simulink model "clutch"  (R2020a)
settings: Solver=ode3  StartTime=0.0  StopTime=30  FixedStep=1e-3  RelTol=1e-3
undefined symbols (not defined in the file or in its folder): be, bv, Ie, Iv, Kd, Ki, Kp, kv, Tclmax
libraries: simulink x2
settings Model: Creator=User  LastModifiedBy=User
settings SolverCC: ZeroCrossAlgorithm=Adaptive
settings DebuggingCC: IgnoredZcDiagnostic=none

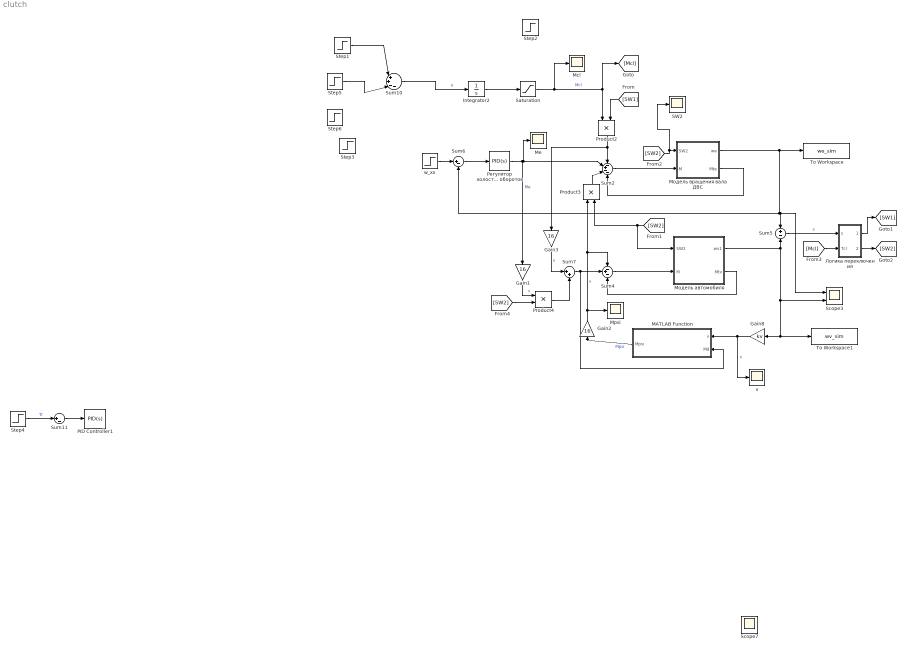
== system clutch ==
  Gain1 : Gain  Gain=16
  Gain2 : Gain  Gain=16
  Gain3 : Gain  Gain=16
  Gain8 : Gain  Gain=kv
  Integrator2 : Integrator
  MATLAB Function : MATLAB Function  TreatAsAtomicUnit=on
  Mcl : Scope
  Me : Scope
  Mpsi : Scope
  PID Controller1 : simulink/Continuous/PID Controller  Controller=PID  Form=Parallel  TimeDomain=Continuous-time  UseExternalTs=off  SampleTime=-1  IntegratorMethod=Forward Euler  FilterMethod=Forward Euler  ControllerParametersSource=internal  P=Kp  I=Ki  D=Kd  UseFilter=on  N=100  TunerSelectOption=Transfer Function Based (PID Tuner App)  InitialConditionSource=internal  InitialConditionForIntegrator=0  InitialConditionForFilter=0  DifferentiatorICPrevScaledInput=0  ExternalReset=none  TrackingMode=off  Kt=1  LimitOutput=off  UpperSaturationLimit=inf  LowerSaturationLimit=0  LinearizeAsGain=on  AntiWindupMode=none  Kb=1  POutMin=[]  POutMax=[]  IOutMin=[]  IOutMax=[]  DOutMin=[]  DOutMax=[]  NOutMin=[]  NOutMax=[]  SumOutMin=[]  SumOutMax=[]  SaturationOutMin=[]  SaturationOutMax=[]  PParamMin=[]  PParamMax=[]  IParamMin=[]  IParamMax=[]  DParamMin=[]  DParamMax=[]  NParamMin=[]  NParamMax=[]  KbParamMin=[]  KbParamMax=[]  KtParamMin=[]  KtParamMax=[]  KbOutMin=[]  KbOutMax=[]  KtOutMin=[]  KtOutMax=[]  IntegratorOutMin=[]  IntegratorOutMax=[]  FilterOutMin=[]  FilterOutMax=[]  SumI1OutMin=[]  SumI1OutMax=[]  SumI2OutMin=[]  SumI2OutMax=[]  SumI3OutMin=[]  SumI3OutMax=[]  SumI4OutMin=[]  SumI4OutMax=[]  SumDOutMin=[]  SumDOutMax=[]  DifferentiatorOutMin=[]  DifferentiatorOutMax=[]  FilterDiffOutCoefMin=[]  FilterDiffOutCoefMax=[]  ReciprocalOutMin=[]  ReciprocalOutMax=[]  SumDenOutMin=[]  SumDenOutMax=[]  SumNumOutMin=[]  SumNumOutMax=[]  DivideOutMin=[]  DivideOutMax=[]  UdiffTsProdOutMin=[]  UdiffTsProdOutMax=[]  NTsProdOutMin=[]  NTsProdOutMax=[]  UintegralTsProdOutMin=[]  UintegralTsProdOutMax=[]  UngainTsProdOutMin=[]  UngainTsProdOutMax=[]  IntegratorContinuousStateAttributes=''  IntegratorStateMustResolveToSignalObject=off  IntegratorRTWStateStorageClass=Auto  FilterContinuousStateAttributes=''  FilterStateMustResolveToSignalObject=off  FilterRTWStateStorageClass=Auto  ParallelPVariant=InternalParameters  IdealPVariant=Disabled  IVariant=InternalParameters  DVariant=InternalParameters  IntegratorVariant=Continuous  SatVariant=Disabled  AWVariant=Passthrough  PCopyVariant=Disabled  TRVariant=Disabled  FdbkBlocksVariant=Forward  IdealPFdbkVariant=Disabled  SatFdbkVariant=Disabled  DerivativeFilterVariant=ContFilter  NVariant=InternalParameters  NCopyVariant=Disabled  FilterICVariant=InternalICsFilter  IntegratorICVariant=InternalICs  ExternalResetVariant=Disabled  TRSumVariant=Passthrough  SumFdbkVariant=Disabled  SumVariant=Sum_PID  TsampFilterVariant=InternalTs  TsampNgainVariant=Passthrough  TsampIntegralVariant=Passthrough
  Product2 : Product
  Product3 : Product
  Product4 : Product
  SW2 : Scope
  Saturation : Saturate  UpperLimit=Tclmax  LowerLimit=0
  Scope3 : Scope  NumInputPorts=2
  Scope7 : Scope
  Step1 : Step  Time=2.9  After=50/2  SampleTime=0
  Step2 : Step  Time=2.9  After=50/2  SampleTime=0
  Step3 : Step  Time=17  After=100/1  SampleTime=0
  Step4 : Step  Time=5  After=6  SampleTime=0
  Step5 : Step  Time=10  After=1000/1  SampleTime=0
  Step6 : Step  Time=12  After=100/1  SampleTime=0
  Sum10 : Sum  Inputs=|++--
  Sum11 : Sum  Inputs=|+-
  Sum2 : Sum  Inputs=-+--
  Sum4 : Sum  Inputs=-+-
  Sum5 : Sum  Inputs=+|-
  Sum6 : Sum  Inputs=|+-
  Sum7 : Sum  Inputs=|++
  To Workspace : ToWorkspace  VariableName=we_sim  SaveFormat=Timeseries  SampleTime=-1
  To Workspace1 : ToWorkspace  VariableName=wv_sim  SaveFormat=Timeseries  SampleTime=-1
  v : Scope
  w_xx : Step  Time=10  Before=750  After=750  SampleTime=0
  Логика переключения : Subsystem
  Модель автомобиля : Subsystem
  Модель вращения вала ДВС : Subsystem
  Регулятор холостых оборотов : simulink/Continuous/PID Controller  Controller=PID  Form=Parallel  TimeDomain=Continuous-time  UseExternalTs=off  SampleTime=-1  IntegratorMethod=Forward Euler  FilterMethod=Forward Euler  ControllerParametersSource=internal  P=0.5  I=1  D=0  UseFilter=on  N=100  TunerSelectOption=Transfer Function Based (PID Tuner App)  InitialConditionSource=internal  InitialConditionForIntegrator=20  InitialConditionForFilter=0  DifferentiatorICPrevScaledInput=0  ExternalReset=none  TrackingMode=off  Kt=1  LimitOutput=off  UpperSaturationLimit=inf  LowerSaturationLimit=0  LinearizeAsGain=on  AntiWindupMode=none  Kb=1  POutMin=[]  POutMax=[]  IOutMin=[]  IOutMax=[]  DOutMin=[]  DOutMax=[]  NOutMin=[]  NOutMax=[]  SumOutMin=[]  SumOutMax=[]  SaturationOutMin=[]  SaturationOutMax=[]  PParamMin=[]  PParamMax=[]  IParamMin=[]  IParamMax=[]  DParamMin=[]  DParamMax=[]  NParamMin=[]  NParamMax=[]  KbParamMin=[]  KbParamMax=[]  KtParamMin=[]  KtParamMax=[]  KbOutMin=[]  KbOutMax=[]  KtOutMin=[]  KtOutMax=[]  IntegratorOutMin=[]  IntegratorOutMax=[]  FilterOutMin=[]  FilterOutMax=[]  SumI1OutMin=[]  SumI1OutMax=[]  SumI2OutMin=[]  SumI2OutMax=[]  SumI3OutMin=[]  SumI3OutMax=[]  SumI4OutMin=[]  SumI4OutMax=[]  SumDOutMin=[]  SumDOutMax=[]  DifferentiatorOutMin=[]  DifferentiatorOutMax=[]  FilterDiffOutCoefMin=[]  FilterDiffOutCoefMax=[]  ReciprocalOutMin=[]  ReciprocalOutMax=[]  SumDenOutMin=[]  SumDenOutMax=[]  SumNumOutMin=[]  SumNumOutMax=[]  DivideOutMin=[]  DivideOutMax=[]  UdiffTsProdOutMin=[]  UdiffTsProdOutMax=[]  NTsProdOutMin=[]  NTsProdOutMax=[]  UintegralTsProdOutMin=[]  UintegralTsProdOutMax=[]  UngainTsProdOutMin=[]  UngainTsProdOutMax=[]  IntegratorContinuousStateAttributes=''  IntegratorStateMustResolveToSignalObject=off  IntegratorRTWStateStorageClass=Auto  FilterContinuousStateAttributes=''  FilterStateMustResolveToSignalObject=off  FilterRTWStateStorageClass=Auto  ParallelPVariant=InternalParameters  IdealPVariant=Disabled  IVariant=InternalParameters  DVariant=InternalParameters  IntegratorVariant=Continuous  SatVariant=Disabled  AWVariant=Passthrough  PCopyVariant=Disabled  TRVariant=Disabled  FdbkBlocksVariant=Forward  IdealPFdbkVariant=Disabled  SatFdbkVariant=Disabled  DerivativeFilterVariant=ContFilter  NVariant=InternalParameters  NCopyVariant=Disabled  FilterICVariant=InternalICsFilter  IntegratorICVariant=InternalICs  ExternalResetVariant=Disabled  TRSumVariant=Passthrough  SumFdbkVariant=Disabled  SumVariant=Sum_PID  TsampFilterVariant=InternalTs  TsampNgainVariant=Passthrough  TsampIntegralVariant=Passthrough
  wires:
  Sum10/1 -> Integrator2/1  "u"
  Product3/1 -> Sum2/3
  ? -> Sum11/2
  [Mcl] -> Логика переключения/2(Tcl)
  Модель автомобиля/1(wv1) -> Scope3/2, To Workspace1/1, Gain8/1, Sum5/2
  Sum4/1 -> Модель автомобиля/2(M)
  Модель вращения вала ДВС/1(we) -> Scope3/1, Sum5/1, Sum6/2, To Workspace/1
  [SW2] -> Модель автомобиля/1(SW2), Product3/2
  Saturation/1 -> Mcl/1, [Mcl], Product2/1  "Mcl"
  Sum2/1 -> Модель вращения вала ДВС/2(M)
  MATLAB Function/1(Mpsi) -> Gain2/1  "Mpsi"
  Sum11/1 -> PID Controller1/1
  [SW1] -> Product2/2
  Gain8/1 -> MATLAB Function/1(v), v/1  "v"
  [SW2] -> Product4/2
  Логика переключения/1(SW1) -> [SW1]
  Sum5/1 -> Логика переключения/1(s)  "s"
  Логика переключения/2(SW2) -> [SW2]
  [SW2] -> SW2/1, Модель вращения вала ДВС/1(SW2)
  Step5/1 -> Sum10/3
  Step4/1 -> Sum11/1  "Tr"
  Sum7/1 -> MATLAB Function/2(Md), Sum4/2
  Регулятор холостых оборотов/1 -> Sum2/2, Me/1, Gain1/1  "Me"
  Product2/1 -> Gain3/1, Sum2/1
  Sum6/1 -> Регулятор холостых оборотов/1
  Product4/1 -> Sum7/2
  Integrator2/1 -> Saturation/1
  w_xx/1 -> Sum6/1
  Модель автомобиля/2(Mtv) -> Sum4/3
  Модель вращения вала ДВС/2(Mte) -> Sum2/4
  Gain1/1 -> Product4/1  "v"
  Gain2/1 -> Mpsi/1, Sum4/1, Product3/1  "v"
  Step1/1 -> Sum10/1
  Gain3/1 -> Sum7/1  "v"

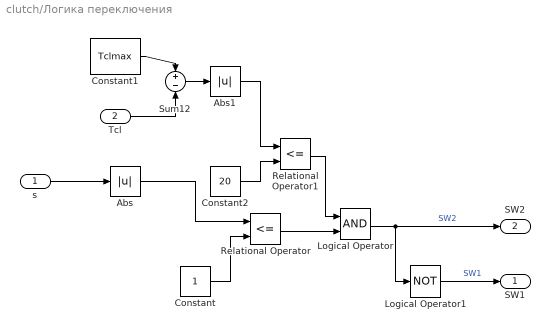
== system clutch/Логика переключения ==
  s : Inport
  Tcl : Inport  Port=2
  Abs : Abs
  Abs1 : Abs
  Constant : Constant
  Constant1 : Constant  Value=Tclmax
  Constant2 : Constant  Value=20
  Logical Operator : Logic  AllPortsSameDT=off  OutDataTypeStr=boolean
  Logical Operator1 : Logic  Operator=NOT  AllPortsSameDT=off  OutDataTypeStr=boolean
  Relational Operator : RelationalOperator  Operator=<=  OutDataTypeStr=boolean  RndMeth=Simplest
  Relational Operator1 : RelationalOperator  Operator=<=  OutDataTypeStr=boolean  RndMeth=Simplest
  Sum12 : Sum  Inputs=+|-
  SW1 : Outport
  SW2 : Outport  Port=2
  wires:
  Constant2/1 -> Relational Operator1/2
  Tcl/1 -> Sum12/2
  Relational Operator/1 -> Logical Operator/2
  Constant1/1 -> Sum12/1
  Logical Operator/1 -> Logical Operator1/1, SW2/1  "SW2"
  Abs1/1 -> Relational Operator1/1
  Relational Operator1/1 -> Logical Operator/1
  Abs/1 -> Relational Operator/1
  Constant/1 -> Relational Operator/2
  Sum12/1 -> Abs1/1
  s/1 -> Abs/1
  Logical Operator1/1 -> SW1/1  "SW1"

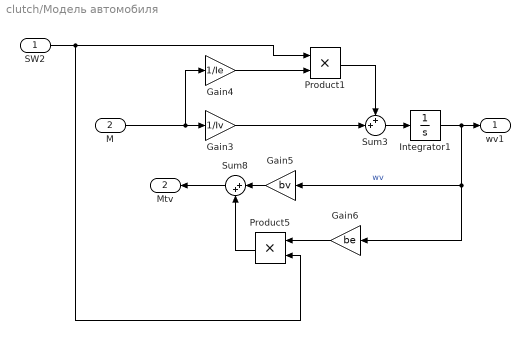
== system clutch/Модель автомобиля ==
  SW2 : Inport
  M : Inport  Port=2
  Gain3 : Gain  Gain=1/Iv
  Gain4 : Gain  Gain=1/Ie
  Gain5 : Gain  Gain=bv
  Gain6 : Gain  Gain=be
  Integrator1 : Integrator
  Product1 : Product
  Product5 : Product
  Sum3 : Sum  Inputs=++|
  Sum8 : Sum  Inputs=|++
  wv1 : Outport
  Mtv : Outport  Port=2
  wires:
  M/1 -> Gain4/1, Gain3/1
  Sum3/1 -> Integrator1/1
  Gain4/1 -> Product1/2
  Gain3/1 -> Sum3/2
  Product1/1 -> Sum3/1
  Gain6/1 -> Product5/1
  Product5/1 -> Sum8/2
  Gain5/1 -> Sum8/1
  SW2/1 -> Product1/1, Product5/2
  Integrator1/1 -> Gain5/1, Gain6/1, wv1/1  "wv"
  Sum8/1 -> Mtv/1

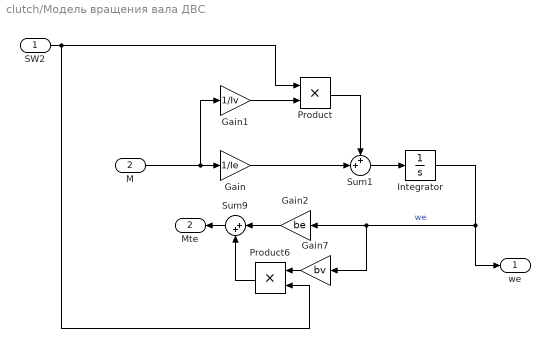
== system clutch/Модель вращения вала ДВС ==
  SW2 : Inport
  M : Inport  Port=2
  Gain : Gain  Gain=1/Ie
  Gain1 : Gain  Gain=1/Iv
  Gain2 : Gain  Gain=be
  Gain7 : Gain  Gain=bv
  Integrator : Integrator  InitialCondition=750
  Product : Product
  Product6 : Product
  Sum1 : Sum  Inputs=++|
  Sum9 : Sum  Inputs=|++
  we : Outport
  Mte : Outport  Port=2
  wires:
  Gain2/1 -> Sum9/1
  Gain7/1 -> Product6/1
  Gain1/1 -> Product/2
  Product/1 -> Sum1/1
  Gain/1 -> Sum1/2
  Integrator/1 -> we/1, Gain2/1, Gain7/1  "we"
  Sum1/1 -> Integrator/1
  M/1 -> Gain1/1, Gain/1
  Product6/1 -> Sum9/2
  SW2/1 -> Product6/2, Product/1
  Sum9/1 -> Mte/1

== matlab function clutch/MATLAB Function ==
  data: v input; Mpsi output; Md input
function Mpsi = RoadResistance(v,Md)

if v == 0
    if abs(Md) < 14.45
        
        Mpsi = Md;
    else
        Mpsi = 14.45;
    end
    
else
   Mpsi = 14.45*sign(v)+2.386*v; 
end
    
end
